simulink model "hw2sim1"  (R2024b)
settings: Solver=VariableStepAuto  StartTime=0.0  StopTime=10.0  RelTol=1e-3
settings Model: Creator=JTerr  LastModifiedBy=JTerr

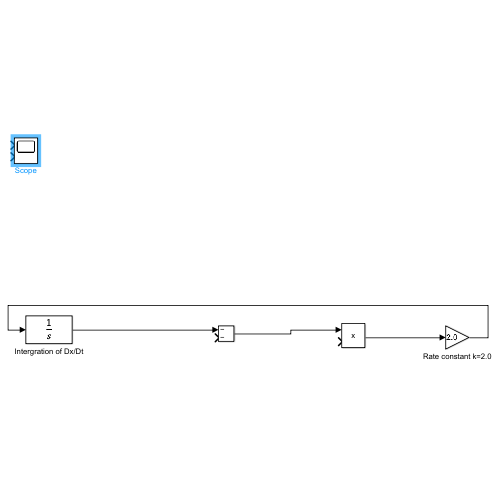
[thumbnail: Simulink's stored preview of the top-level diagram]
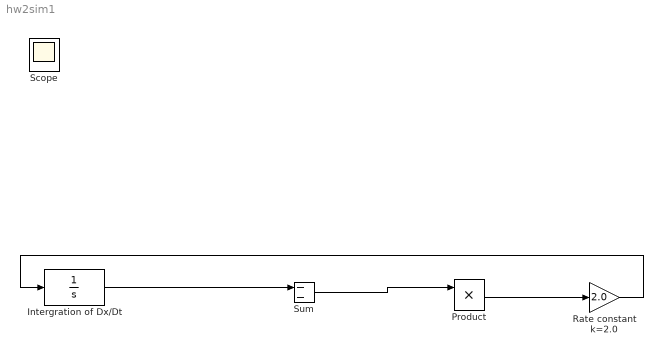
== system hw2sim1 ==
  Intergration of Dx/Dt : Integrator
  Product : Product  OutMin=6.5  OutMax=10.5
  Rate constant k=2.0 : Gain  Gain=2.0
  Scope : Scope  NumInputPorts=2
  Sum : Sum  Inputs=--  OutMin=6.5  OutMax=10.5
  wires:
  Intergration of Dx/Dt/1 -> Sum/1
  Sum/1 -> Product/1
  Product/1 -> Rate constant k=2.0/1
  Rate constant k=2.0/1 -> Intergration of Dx/Dt/1
